simulink model "Linear_Trajectory_Tracking_xd_y_d_Simulink"  (R2025b)
settings: Solver=VariableStepAuto  StartTime=0.0  StopTime=10.0  RelTol=1e-3
values from neighbouring files (symbols this model uses):
  k_v = 0.1    [constants.m]
  k_w = 0.1    [constants.m]
settings Model: Creator=emica  LastModifiedBy=jayamalsigera

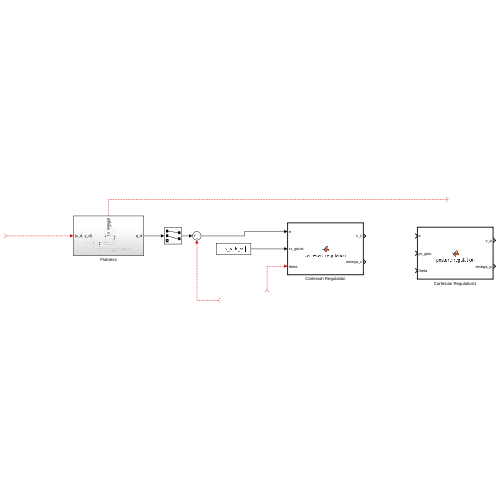
[thumbnail: Simulink's stored preview of the top-level diagram]
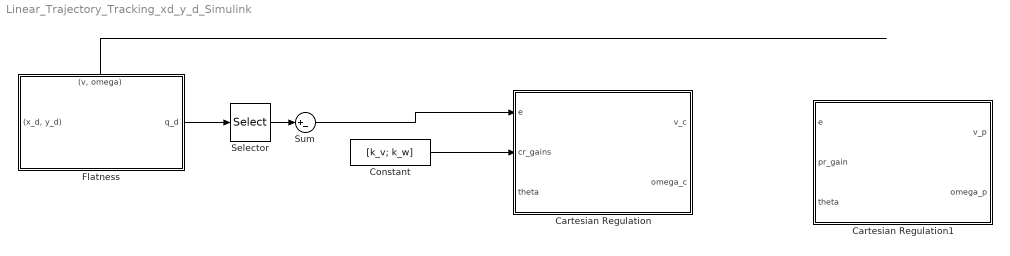
== system Linear_Trajectory_Tracking_xd_y_d_Simulink ==
  Cartesian Regulation : MATLAB Function  TreatAsAtomicUnit=on
  Cartesian Regulation1 : MATLAB Function  TreatAsAtomicUnit=on
  Constant : Constant  Value=[k_v; k_w]
  Flatness : Subsystem
      settings: PortSchema="{\"entries\":[{\"content\":{\"sides\":[{\"content\":{\"connectorIds\":[\"In1\"]},\"type\":\"ConnectorPlacement.EquallySpacedRectSide\",\"uuid\":\"41995734-3ce3-4477-88f1-3d8a67c46faa\"},{\"content\":{\"connectorIds\":[\"Out1\"],\"side\":\"RIGHT\"},\"type\":\"ConnectorPlacement.EquallySpacedRectSide\",\"uuid\":\"c3b5199c-2463-46a8-a170-afba7407f7e0\"},{\"content\":{\"connectorIds\":[\"Out2\"],\"side\":\"TOP\"},\"type\":\"ConnectorPlacement.EquallySpacedRectSide\",\"uuid\":\"c43b9e41-3f4c-44b9-970b-a1c148dbbedd\"}]},\"type\":\"ConnectorPlacement.EquallySpacedConnector\",\"uuid\":\"73da9ae3-dc7e-4d3b-ad2c-470943e261f5\"}],\"packageUris\":[\"http://schema.mathworks.com/mf0/Connector/R2020b\"],\"version\":\"1.0\"}"
  Selector : Selector  InputPortWidth=3  IndexOptions=Index vector (dialog)  Indices=[1 2]  OutputSizes=1
  Sum : Sum  Inputs=|+-
  wires:
  ? -> Flatness/1("(x_d, y_d)")
  Selector/1 -> Sum/1
  Flatness/1(q_d) -> Selector/1
  Flatness/2("(v, omega)") -> ?
  Constant/1 -> Cartesian Regulation/2(cr_gains)
  ? -> Sum/2
  Sum/1 -> Cartesian Regulation/1(e)
  ? -> Cartesian Regulation/3(theta)

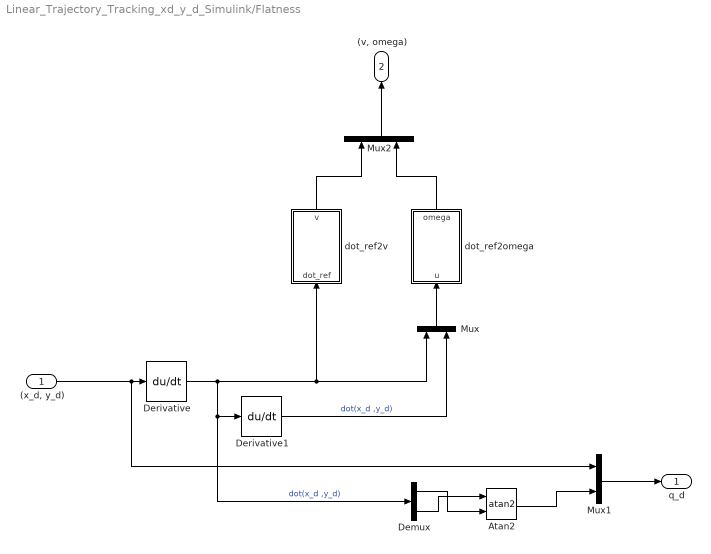
== system Linear_Trajectory_Tracking_xd_y_d_Simulink/Flatness ==
  "(x_d, y_d)" : Inport
  Atan2 : Trigonometry  Operator=atan2
  Demux : Demux  Outputs=2
  Derivative : Derivative
  Derivative1 : Derivative
  Mux : Mux  Inputs=2
  Mux1 : Mux  Inputs=2
  Mux2 : Mux  Inputs=2
  dot_ref2omega : MATLAB Function  TreatAsAtomicUnit=on
  dot_ref2v : MATLAB Function  TreatAsAtomicUnit=on
  q_d : Outport
  "(v, omega)" : Outport  Port=2
  wires:
  dot_ref2omega/1(omega) -> Mux2/2
  Mux1/1 -> q_d/1
  Mux/1 -> dot_ref2omega/1(u)
  Demux/1 -> Atan2/2
  dot_ref2v/1(v) -> Mux2/1
  Mux2/1 -> "(v, omega)"/1
  Atan2/1 -> Mux1/2
  Demux/2 -> Atan2/1
  Derivative1/1 -> Mux/2  "dot(x_d ,y_d)"
  "(x_d, y_d)"/1 -> Mux1/1, Derivative/1
  Derivative/1 -> Mux/1, dot_ref2v/1(dot_ref), Demux/1, Derivative1/1  "dot(x_d ,y_d)"

== matlab function Linear_Trajectory_Tracking_xd_y_d_Simulink/Flatness/dot_ref2omega ==
  data: u input; omega output
function omega = fcn(u)
    dot_x = u(1);
    dot_y = u(2);
    ddot_x = u(3);
    ddot_y = u(4);

    omega = (dot_x*ddot_y - dot_y*ddot_x) / (dot_x^2 + dot_y^2);

== matlab function Linear_Trajectory_Tracking_xd_y_d_Simulink/Flatness/dot_ref2v ==
  data: dot_ref input; v output
function v = fcn(dot_ref)
    dot_x = dot_ref(1);
    dot_y = dot_ref(2);

    v = sqrt(dot_x^2 + dot_y^2);

== matlab function Linear_Trajectory_Tracking_xd_y_d_Simulink/Cartesian Regulation ==
  data: e input; v_c output; cr_gains input; omega_c output; theta input
function [v_c, omega_c] = cartesian_regulation(e, cr_gains, theta)

e_x = e(1);
e_y = e(2);

% Gains
k_v = cr_gains(1);
k_w = cr_gains(2);

% Projection of error on sagittal axis
e_n = e_x*cos(theta) + e_y*sin(theta);

% Angle to the target
alpha = atan2(e_y, e_x);

% Orientation error
delta = wrapToPi(alpha - theta);

% Cartesian regulation laws
v_c = k_v * e_n;
omega_c = k_w * delta;


end

== matlab function Linear_Trajectory_Tracking_xd_y_d_Simulink/Cartesian Regulation1 ==
  data: e input; v_p output; pr_gain input; omega_p output; theta input
function [v_p, omega_p] = posture_regulation(e, pr_gain, theta)

e_x = e(1);
e_y = e(2);

% Gains
k_delta = pr_gain;

% length of error vector 
rho = sqrt(omega = ...
    k_w * gamma + ...
    k_v * sinc_term * cos(gamma) * (gamma + k_delta * delta);x^2 + y^2);

% Angles Gamma and Delta
gamma = atan2(y, x) + pi - theta;
gamma = wrapToPi(gamma);

delta = wrapToPi(gamma + theta);

% Posture regulation laws
v_p = k_v * rho * cos(gamma);
omega_p = k_w * gamma + k_v * sinc_term * cos(gamma) * (gamma + k_delta * delta);

end
